simulink model "yaw_loop"  (Simulink 8.2)
settings: Solver=ode45  StartTime=0.0  StopTime=200  RelTol=1e-3
undefined symbols (not defined in the file): P
settings Model: Creator=paul  LastModifiedBy=paul
settings DataIOCC: SignalLoggingSaveFormat=Dataset
settings OptimizationCC: ExpressionDepthLimit=128
settings DebuggingCC: FcnCallInpInsideContextMsg=EnableAllAsError  StateNameClashWarn=none
settings GRTTargetCC: CombineOutputUpdateFcns=on  GRTInterface=off

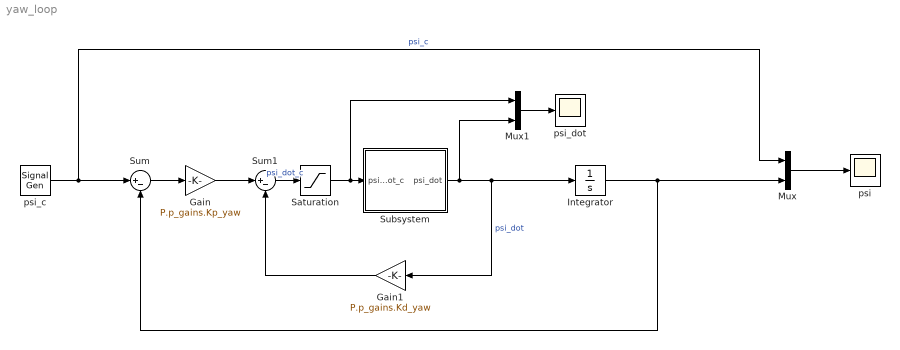
== system yaw_loop ==
  Gain : Gain  Gain=P.p_gains.Kp_yaw
  Gain1 : Gain  Gain=P.p_gains.Kd_yaw
  Integrator : Integrator
  Mux : Mux  Inputs=2
  Mux1 : Mux  Inputs=2
  Saturation : Saturate  UpperLimit=P.yaw_rate_c_max  LowerLimit=-P.yaw_rate_c_max
  Subsystem : Subsystem
  Sum : Sum  Inputs=|+-
  Sum1 : Sum  Inputs=|+-
  psi : Scope
  psi_c : SignalGenerator  WaveForm=square  Amplitude=45*pi/180  Frequency=0.05  Units=rad/sec
  psi_dot : Scope
  wires:
  Mux/1 -> psi/1
  psi_c/1 -> Sum/1, Mux/1  "psi_c"
  Subsystem/1(psi_dot) -> Mux1/2, Gain1/1, Integrator/1  "psi_dot"
  Sum/1 -> Gain/1
  Sum1/1 -> Saturation/1  "psi_dot_c"
  Gain/1 -> Sum1/1
  Gain1/1 -> Sum1/2
  Integrator/1 -> Sum/2, Mux/2
  Mux1/1 -> psi_dot/1
  Saturation/1 -> Mux1/1, Subsystem/1(psi_dot_c)

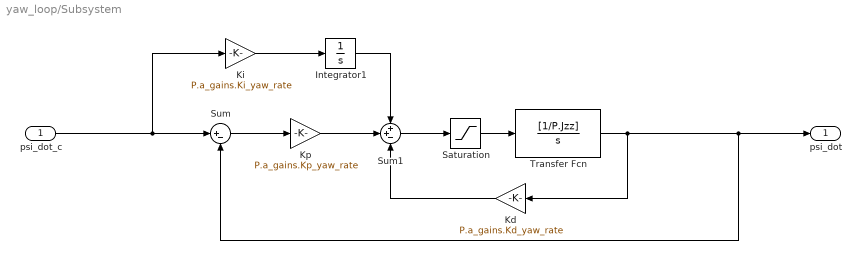
== system yaw_loop/Subsystem ==
  psi_dot_c : Inport
  Integrator1 : Integrator
  Kd : Gain  Gain=P.a_gains.Kd_yaw_rate
  Ki : Gain  Gain=P.a_gains.Ki_yaw_rate
  Kp : Gain  Gain=P.a_gains.Kp_yaw_rate
  Saturation : Saturate  UpperLimit=P.T_psi_max  LowerLimit=-P.T_psi_max
  Sum : Sum  Inputs=|+-
  Sum1 : Sum  Inputs=++-
  Transfer Fcn : TransferFcn  Numerator=[1/P.Jzz]  Denominator=[1 0]
  psi_dot : Outport
  wires:
  Saturation/1 -> Transfer Fcn/1
  Transfer Fcn/1 -> psi_dot/1, Sum/2, Kd/1
  Kp/1 -> Sum1/2
  Ki/1 -> Integrator1/1
  Sum1/1 -> Saturation/1
  Sum/1 -> Kp/1
  Integrator1/1 -> Sum1/1
  Kd/1 -> Sum1/3
  psi_dot_c/1 -> Ki/1, Sum/1
